simulink model "carBrakeSoln"  (R2015a)
settings: Solver=ode23t  StartTime=0.0  StopTime=50  RelTol=1e-3  AbsTol=1e-3
libraries: nesl_utility x20, fl_lib x18, sdl_lib x11, simulink x1
settings Model: FPTRunName=Active  CovSFcnEnable=off  ExtModeAutoUpdateStatusClock=off  Creator=MathWorks  LastModifiedBy=sseshadr
settings SolverCC: ZcThreshold=0  ZeroCrossAlgorithm=Adaptive
settings DataIOCC: SignalLoggingSaveFormat=ModelDataLogs  SaveOutput=off  SignalLogging=off  DSMLogging=off  SaveTime=off
settings OptimizationCC: ExpressionDepthLimit=2147483647  InitFltsAndDblsToZero=on  BufferReusableBoundary=off
settings DebuggingCC: SaveWithParameterizedLinksMsg=none  UnderspecifiedInitializationDetection=Classic  MergeDetectMultiDrivingBlocksExec=none  SignalResolutionControl=TryResolveAllWithWarning  MultiTaskDSMMsg=warning  MultiTaskCondExecSysMsg=none  SigSpecEnsureSampleTimeMsg=none  FcnCallInpInsideContextMsg=UseLocalSettings  BusObjectLabelMismatch=none  StateNameClashWarn=warning
settings HardwareCC: TargetLongLongMode=on  TargetEndianess=LittleEndian  TargetHWDeviceType=MATLAB Host  ProdEqTarget=off
settings GRTTargetCC: CombineOutputUpdateFcns=off  GRTInterface=on

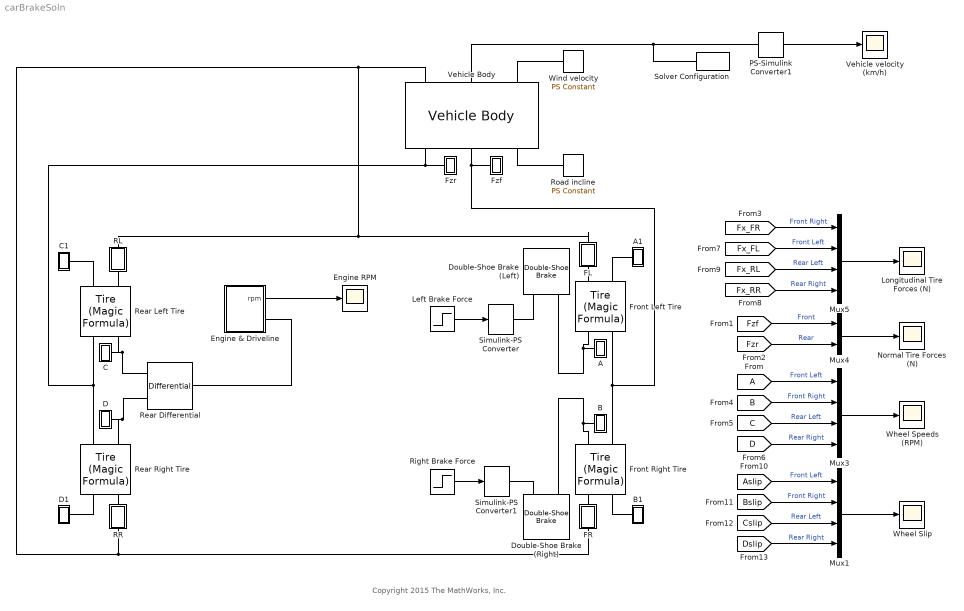
== system carBrakeSoln ==
  note: Copyright 2015 The MathWorks, Inc.
  A : Subsystem
  A1 : Subsystem
  B : Subsystem
  B1 : Subsystem
  C : Subsystem
  C1 : Subsystem
  D : Subsystem
  D1 : Subsystem
  Double-Shoe Brake (Left) : sdl_lib/Brakes & Detents/Rotational/Double-Shoe Brake  r_drum=200 mm  r_act=150 mm  r_pin=125 mm  theta_pin=15 deg  theta_0=5 deg  theta_shoe=120 deg  mu_visc=.01 N*m/(rad/s)  mu=0.3  w_thr=0.01 rad/s
  Double-Shoe Brake (Right) : sdl_lib/Brakes & Detents/Rotational/Double-Shoe Brake  r_drum=200 mm  r_act=150 mm  r_pin=125 mm  theta_pin=15 deg  theta_0=5 deg  theta_shoe=120 deg  mu_visc=.01 N*m/(rad/s)  mu=0.3  w_thr=0.01 rad/s
  Engine RPM : Scope
      settings: TimeRange=30  YMin=600  YMax=1800  SaveName=ScopeData3
  Engine & Driveline : Subsystem
  FL : Subsystem
  FR : Subsystem
  Front Left Tire : sdl_lib/Tires & Vehicles/Tire (Magic Formula)  parameterization=1  F_z1=3000 N  F_x1=3500 N  kappa1=10  B_m=10  C_m=1.9  D_m=1  E_m=0.97  fz0=4e+3 N  p_Cx=1.685  p_Dx=[ 1.21 -0.037 ]  p_Ex=[ 0.344 0.095 -0.02 0 ]  p_Kx=[ 21.51 -0.163 0.245 ]  p_Hx=[ -0.002 0.002 ]  p_Vx=[ 0 0 ]  v_tr_thr=0.1 m/s  r_e=16*2.54/100 m  model_compliance=1  stiffness=200000 N/m  damping=1000 N/(m/s)  model_inertia=1  inertia=4.129 kg*m^2  initial_velocity=0 rpm  model_resistance=1  resistance_model=1  coeff=0.015  p_tire=250e3 Pa  alpha=-0.003  beta=0.97  coeff_a=84e-4  coeff_b=6.2e-4 s/m  coeff_c=1.6e-4 s^2/m^2  v_thr=1e-3 m/s
  Front Right Tire : sdl_lib/Tires & Vehicles/Tire (Magic Formula)  parameterization=1  F_z1=3000 N  F_x1=3500 N  kappa1=10  B_m=10  C_m=1.9  D_m=1  E_m=0.97  fz0=4e+3 N  p_Cx=1.685  p_Dx=[ 1.21 -0.037 ]  p_Ex=[ 0.344 0.095 -0.02 0 ]  p_Kx=[ 21.51 -0.163 0.245 ]  p_Hx=[ -0.002 0.002 ]  p_Vx=[ 0 0 ]  v_tr_thr=0.1 m/s  r_e=16*2.54/100 m  model_compliance=1  stiffness=200000 N/m  damping=1000 N/(m/s)  model_inertia=1  inertia=4.129 kg*m^2  initial_velocity=0 rpm  model_resistance=1  resistance_model=1  coeff=0.015  p_tire=250e3 Pa  alpha=-0.003  beta=0.97  coeff_a=84e-4  coeff_b=6.2e-4 s/m  coeff_c=1.6e-4 s^2/m^2  v_thr=1e-3 m/s
  Fzf : Subsystem
  Fzr : Subsystem
  Left Brake Force : Step  Time=30  After=1000  SampleTime=0
      settings: AttributesFormatString=Brake on @ %<Time> s
  Longitudinal Tire Forces (N) : Scope
      settings: ShowLegends=on  TimeRange=50  YMin=-1500  YMax=3500  SaveName=ScopeData4
  Mux1 : Mux
  Mux3 : Mux
  Mux4 : Mux  Inputs=2
  Mux5 : Mux
  Normal Tire Forces (N) : Scope
      settings: ShowLegends=on  TimeRange=50  YMin=3200  YMax=3900  SaveName=ScopeData2
  PS-Simulink Converter1 : nesl_utility/PS-Simulink Converter  PhysicalDomain=network_engine_domain  SubClassName=ps_output  LeftPortType=input  RightPortType=output  PseudoPeriodic=off  Frequencies=[]  Unit=km/hr  AffineConversion=off
  RL : Subsystem
  RR : Subsystem
  Rear Differential : sdl_lib/Gears/Differential  driveshaft_location=2  cd_ratio=4  friction_model=1  efficiency=[ 0.85 0.92 ]  mu_visc=[ 0 0 ] N*m/(rad/s)  w_thr=[ 0.01 0.01 ] rad/s  temperature_TLU=[ 280 300 320 ] K  efficiency_ss_TLU=[ 0.95 0.9 0.85 ]  efficiency_cd_TLU=[ 0.95 0.9 0.85 ]  thermal_mass=50 J/K  T_init=300 K
  Rear Left Tire : sdl_lib/Tires & Vehicles/Tire (Magic Formula)  parameterization=1  F_z1=3000 N  F_x1=3500 N  kappa1=10  B_m=10  C_m=1.9  D_m=1  E_m=0.97  fz0=4e+3 N  p_Cx=1.685  p_Dx=[ 1.21 -0.037 ]  p_Ex=[ 0.344 0.095 -0.02 0 ]  p_Kx=[ 21.51 -0.163 0.245 ]  p_Hx=[ -0.002 0.002 ]  p_Vx=[ 0 0 ]  v_tr_thr=0.1 m/s  r_e=16*2.54/100 m  model_compliance=1  stiffness=200000 N/m  damping=1000 N/(m/s)  model_inertia=1  inertia=4.129 kg*m^2  initial_velocity=0 rpm  model_resistance=1  resistance_model=1  coeff=0.015  p_tire=250e3 Pa  alpha=-0.003  beta=0.97  coeff_a=84e-4  coeff_b=6.2e-4 s/m  coeff_c=1.6e-4 s^2/m^2  v_thr=1e-3 m/s
  Rear Right Tire : sdl_lib/Tires & Vehicles/Tire (Magic Formula)  parameterization=1  F_z1=3000 N  F_x1=3500 N  kappa1=10  B_m=10  C_m=1.9  D_m=1  E_m=0.97  fz0=4e+3 N  p_Cx=1.685  p_Dx=[ 1.21 -0.037 ]  p_Ex=[ 0.344 0.095 -0.02 0 ]  p_Kx=[ 21.51 -0.163 0.245 ]  p_Hx=[ -0.002 0.002 ]  p_Vx=[ 0 0 ]  v_tr_thr=0.1 m/s  r_e=16*2.54/100 m  model_compliance=1  stiffness=200000 N/m  damping=1000 N/(m/s)  model_inertia=1  inertia=4.129 kg*m^2  initial_velocity=0 rpm  model_resistance=1  resistance_model=1  coeff=0.015  p_tire=250e3 Pa  alpha=-0.003  beta=0.97  coeff_a=84e-4  coeff_b=6.2e-4 s/m  coeff_c=1.6e-4 s^2/m^2  v_thr=1e-3 m/s
  Right Brake Force : Step  Time=30  After=1000  SampleTime=0
      settings: AttributesFormatString=Brake on @ %<Time> s
  Road incline : fl_lib/Physical Signals/Sources/PS Constant  constant=pi*15/180
  Simulink-PS Converter : nesl_utility/Simulink-PS Converter  PhysicalDomain=network_engine_domain  SubClassName=ps_input  LeftPortType=input  RightPortType=output  PseudoPeriodic=off  Frequencies=[]  NoiseDistribution=none  NoiseParameters=[]  Unit=1  AffineConversion=off  InputFiltering=off  SimscapeFilterOrder=1  InputFilterTimeConstant=0.001  UdotUserProvided=1
  Simulink-PS Converter1 : nesl_utility/Simulink-PS Converter  PhysicalDomain=network_engine_domain  SubClassName=ps_input  LeftPortType=input  RightPortType=output  PseudoPeriodic=off  Frequencies=[]  NoiseDistribution=none  NoiseParameters=[]  Unit=1  AffineConversion=off  InputFiltering=off  SimscapeFilterOrder=1  InputFilterTimeConstant=0.001  UdotUserProvided=1
  Solver Configuration : nesl_utility/Solver Configuration  PhysicalDomain=network_engine_domain  SubClassName=solver  LeftPortType=input  RightPortType=generic  Accelerate=off  Tones=[]  Harmonics=[]  SimulateNoise=off  Profile=off  UseLocalSampling=off  EnableSwitchedLinearOptims=on  FrequencyDomain=off  UseCCode=off  RelTol=0.001  AbsTol=1e-06  MinStep=1e-09  ToWorkspace=off  RevertToSquareIcSolve=off  NumHomotopyIterations=100  DoDC=off  ResidualTolerance=1e-9  UseLocalSolver=off  LocalSolverChoice=NE_BACKWARD_EULER_ADVANCER  LocalSolverSampleTime=0.1  DoFixedCost=off  MaxNonlinIter=3  MaxModeIter=2  LinearAlgebra=Sparse  DelaysMemoryBudget=1024  AutomaticFiltering=on  FilteringTimeConstant=0.001
  Vehicle Body : sdl_lib/Tires & Vehicles/Vehicle Body  mass=1500 kg  n_w=2  x_f=1.4 m  x_r=1.6 m  y_c=0.5 m  area=3 m^2  Cd=0.4  v0=0 m/s  g=9.81 m/s^2  rho=1.18 kg/m^3
  Vehicle velocity (km/h) : Scope
      settings: TimeRange=50  YMax=25  SaveName=ScopeData6
  Wheel Slip : Scope
      settings: ShowLegends=on  TimeRange=50  YMin=-0.01  YMax=0.035
  Wheel Speeds (RPM) : Scope
      settings: ShowLegends=on  TimeRange=50  YMin=-20  YMax=140
  Wind velocity : fl_lib/Physical Signals/Sources/PS Constant  constant=0
  wires:
  Engine & Driveline/1(rpm) -> Engine RPM/1
  PS-Simulink Converter1/1 -> Vehicle velocity (km/h)/1
  Left Brake Force/1 -> Simulink-PS Converter/1
  Right Brake Force/1 -> Simulink-PS Converter1/1
  Mux5/1 -> Longitudinal Tire Forces (N)/1
  Mux4/1 -> Normal Tire Forces (N)/1
  Mux3/1 -> Wheel Speeds (RPM)/1
  Mux1/1 -> Wheel Slip/1
  [A] -> Mux3/1  "Front Left"
  [B] -> Mux3/2  "Front Right"
  [C] -> Mux3/3  "Rear Left"
  [D] -> Mux3/4  "Rear Right"
  [Fzf] -> Mux4/1  "Front"
  [Fzr] -> Mux4/2  "Rear"
  [Fx_FR] -> Mux5/1  "Front Right"
  [Fx_FL] -> Mux5/2  "Front Left"
  [Fx_RR] -> Mux5/4  "Rear Right"
  [Fx_RL] -> Mux5/3  "Rear Left"
  [Aslip] -> Mux1/1  "Front Left"
  [Bslip] -> Mux1/2  "Front Right"
  [Cslip] -> Mux1/3  "Rear Left"
  [Dslip] -> Mux1/4  "Rear Right"
  connections:
  Rear Differential/RConn1 -- Rear Left Tire/LConn2 -- C/LConn1
  D/LConn1 -- Rear Right Tire/LConn2 -- Rear Differential/RConn2
  A/LConn1 -- Double-Shoe Brake (Left)/LConn2 -- Front Left Tire/LConn2
  FL/RConn1 -- RL/RConn1 -- RR/RConn1 -- FR/RConn1 -- Vehicle Body/LConn1
  Front Right Tire/LConn1 -- Front Left Tire/LConn1 -- Vehicle Body/RConn2 -- Fzf/LConn1
  Vehicle Body/RConn1 -- Fzr/LConn1 -- Rear Right Tire/LConn1 -- Rear Left Tire/LConn1
  Road incline/RConn1 -- Vehicle Body/RConn3
  Wind velocity/RConn1 -- Vehicle Body/LConn3
  Vehicle Body/LConn2 -- PS-Simulink Converter1/LConn1 -- Solver Configuration/RConn1
  Front Right Tire/RConn2 -- FR/LConn1
  Rear Right Tire/RConn2 -- RR/LConn1
  Front Left Tire/RConn2 -- FL/LConn1
  Rear Left Tire/RConn2 -- RL/LConn1
  Front Left Tire/RConn1 -- A1/LConn1
  Front Right Tire/RConn1 -- B1/LConn1
  Rear Right Tire/RConn1 -- D1/LConn1
  Rear Left Tire/RConn1 -- C1/LConn1
  Double-Shoe Brake (Left)/LConn1 -- Simulink-PS Converter/RConn1
  Double-Shoe Brake (Right)/LConn1 -- Simulink-PS Converter1/RConn1
  Engine & Driveline/RConn1 -- Rear Differential/LConn1
  Front Right Tire/LConn2 -- Double-Shoe Brake (Right)/LConn2 -- B/LConn1

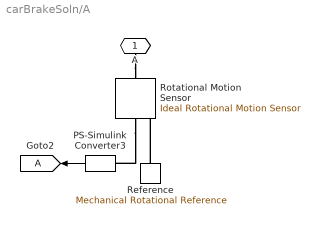
== system carBrakeSoln/A ==
  PS-Simulink Converter3 : nesl_utility/PS-Simulink Converter  PhysicalDomain=network_engine_domain  SubClassName=ps_output  LeftPortType=input  RightPortType=output  PseudoPeriodic=off  Frequencies=[]  Unit=rpm  AffineConversion=off
  Reference : fl_lib/Mechanical/Rotational Elements/Mechanical Rotational Reference
  Rotational Motion Sensor : fl_lib/Mechanical/Mechanical Sensors/Ideal Rotational Motion Sensor  offset=0 rad
  A : PMIOPort  Port=1  Side=Left
  tag scope: A=global
  wires:
  PS-Simulink Converter3/1 -> [A]
  connections:
  Rotational Motion Sensor/RConn2 -- PS-Simulink Converter3/LConn1
  Reference/LConn1 -- Rotational Motion Sensor/RConn1
  A/RConn1 -- Rotational Motion Sensor/LConn1

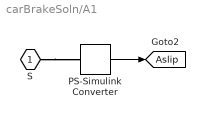
== system carBrakeSoln/A1 ==
  PS-Simulink Converter : nesl_utility/PS-Simulink Converter  PhysicalDomain=network_engine_domain  SubClassName=ps_output  LeftPortType=input  RightPortType=output  PseudoPeriodic=off  Frequencies=[]  Unit=1  AffineConversion=off
  S : PMIOPort  Port=1  Side=Left
  tag scope: Aslip=global
  wires:
  PS-Simulink Converter/1 -> [Aslip]
  connections:
  S/RConn1 -- PS-Simulink Converter/LConn1

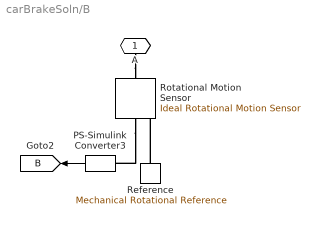
== system carBrakeSoln/B ==
  PS-Simulink Converter3 : nesl_utility/PS-Simulink Converter  PhysicalDomain=network_engine_domain  SubClassName=ps_output  LeftPortType=input  RightPortType=output  PseudoPeriodic=off  Frequencies=[]  Unit=rpm  AffineConversion=off
  Reference : fl_lib/Mechanical/Rotational Elements/Mechanical Rotational Reference
  Rotational Motion Sensor : fl_lib/Mechanical/Mechanical Sensors/Ideal Rotational Motion Sensor  offset=0 rad
  A : PMIOPort  Port=1  Side=Left
  tag scope: B=global
  wires:
  PS-Simulink Converter3/1 -> [B]
  connections:
  A/RConn1 -- Rotational Motion Sensor/LConn1
  Reference/LConn1 -- Rotational Motion Sensor/RConn1
  Rotational Motion Sensor/RConn2 -- PS-Simulink Converter3/LConn1

== system carBrakeSoln/B1 ==
  PS-Simulink Converter : nesl_utility/PS-Simulink Converter  PhysicalDomain=network_engine_domain  SubClassName=ps_output  LeftPortType=input  RightPortType=output  PseudoPeriodic=off  Frequencies=[]  Unit=1  AffineConversion=off
  S : PMIOPort  Port=1  Side=Left
  tag scope: Bslip=global
  wires:
  PS-Simulink Converter/1 -> [Bslip]
  connections:
  S/RConn1 -- PS-Simulink Converter/LConn1

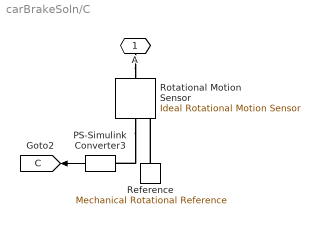
== system carBrakeSoln/C ==
  PS-Simulink Converter3 : nesl_utility/PS-Simulink Converter  PhysicalDomain=network_engine_domain  SubClassName=ps_output  LeftPortType=input  RightPortType=output  PseudoPeriodic=off  Frequencies=[]  Unit=rpm  AffineConversion=off
  Reference : fl_lib/Mechanical/Rotational Elements/Mechanical Rotational Reference
  Rotational Motion Sensor : fl_lib/Mechanical/Mechanical Sensors/Ideal Rotational Motion Sensor  offset=0 rad
  A : PMIOPort  Port=1  Side=Left
  tag scope: C=global
  wires:
  PS-Simulink Converter3/1 -> [C]
  connections:
  Rotational Motion Sensor/RConn2 -- PS-Simulink Converter3/LConn1
  Reference/LConn1 -- Rotational Motion Sensor/RConn1
  A/RConn1 -- Rotational Motion Sensor/LConn1

== system carBrakeSoln/C1 ==
  PS-Simulink Converter : nesl_utility/PS-Simulink Converter  PhysicalDomain=network_engine_domain  SubClassName=ps_output  LeftPortType=input  RightPortType=output  PseudoPeriodic=off  Frequencies=[]  Unit=1  AffineConversion=off
  S : PMIOPort  Port=1  Side=Left
  tag scope: Cslip=global
  wires:
  PS-Simulink Converter/1 -> [Cslip]
  connections:
  S/RConn1 -- PS-Simulink Converter/LConn1

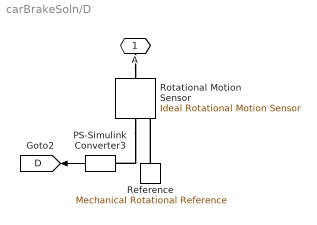
== system carBrakeSoln/D ==
  PS-Simulink Converter3 : nesl_utility/PS-Simulink Converter  PhysicalDomain=network_engine_domain  SubClassName=ps_output  LeftPortType=input  RightPortType=output  PseudoPeriodic=off  Frequencies=[]  Unit=rpm  AffineConversion=off
  Reference : fl_lib/Mechanical/Rotational Elements/Mechanical Rotational Reference
  Rotational Motion Sensor : fl_lib/Mechanical/Mechanical Sensors/Ideal Rotational Motion Sensor  offset=0 rad
  A : PMIOPort  Port=1  Side=Left
  tag scope: D=global
  wires:
  PS-Simulink Converter3/1 -> [D]
  connections:
  A/RConn1 -- Rotational Motion Sensor/LConn1
  Reference/LConn1 -- Rotational Motion Sensor/RConn1
  Rotational Motion Sensor/RConn2 -- PS-Simulink Converter3/LConn1

== system carBrakeSoln/D1 ==
  PS-Simulink Converter : nesl_utility/PS-Simulink Converter  PhysicalDomain=network_engine_domain  SubClassName=ps_output  LeftPortType=input  RightPortType=output  PseudoPeriodic=off  Frequencies=[]  Unit=1  AffineConversion=off
  S : PMIOPort  Port=1  Side=Left
  tag scope: Dslip=global
  wires:
  PS-Simulink Converter/1 -> [Dslip]
  connections:
  S/RConn1 -- PS-Simulink Converter/LConn1

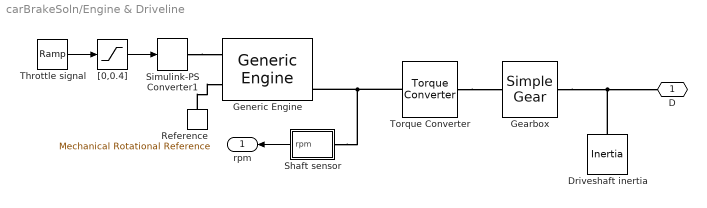
== system carBrakeSoln/Engine & Driveline ==
  Driveshaft inertia : fl_lib/Mechanical/Rotational Elements/Inertia  inertia=12 kg*m^2  w_specify=off  w_priority=High  w=0 rad/s  t_specify=off  t_priority=High  t=0 N*m
  Gearbox : sdl_lib/Gears/Simple Gear  ratio=2  rotation_direction=1  friction_model=1  T_noload=0.1 N*m  T_nom=5 N*m  efficiency_nom=0.8  efficiency=0.8  mu_visc=[ 0 0 ] N*m/(rad/s)  w_thr=0.01 rad/s  temperature_TLU=[ 280 300 320 ] K  load_TLU=[ 1 5 10 ] N*m  efficiency_TLU=[ 0.95 0.9 0.85 ]  efficiency_TLU2=[ 0.85 0.8 0.75; 0.95 0.9 0.85; 0.85 0.8 0.7 ]  thermal_mass=50 J/K  T_init=300 K
  Generic Engine : sdl_lib/Engines/Generic Engine  model_parameterization=1  engine_type=1  P_max=150e3 W  w_P_max=4500 rpm  w_max=6000 rpm  w_min=500 rpm  w_tab=[ 500 1000 2e+3 3e+3 4e+3 5e+3 6e+3 7e+3 ] rpm  trq_tab=[ 380 380 380 380 350 280 200 80 ] N*m  pwr_tab=[ 2e+4 4e+4 7.8e+4 1.2e+5 1.45e+5 1.48e+5 1.25e+5 6e+4 ] W  interp_method=1  model_inertia=1  inertia=0.2 kg*m^2  initial_velocity=800 rpm  model_time_constant=0  time_constant=0.2 s  T0=0  w_thr=100 rpm  idle_speed=0  idle_speed_reference=1000 rpm  tau_controller=1 s  idle_w_thr=1 rpm  fc_model=1  fc_per_rev=25 mg/rev  displaced_volume=400 cm^3  rev_per_cycle=2  fc_w_tab=[ 1000 2e+3 3e+3 4e+3 5e+3 6e+3 ] rpm  fc_trq_tab=[ 0 80 160 200 240 320 360 400 ] N*m  fc_tab=[ 0.5 0.9 1.4 1.6 1.9 2.7 3.4 4.4; 1 1.7 2.7 3.1 3.6 5 6 7.4; 1.4 2.7 4 4.8 5.6 7.5 8.5 10.5; 2 3.6 5.8 6.7 8 10.4 11.7 13.3; 2.5 4.8 7.9 9.4 10.8 14 16.2 18.6; 3.1 6 10.3 11.9 13.8 18.4 22 26.5 ] g/s  bmep_tab=[ 0 250 500 625 750 1000 1.15e+3 1.25e+3 ] kPa  bsfc_tab=[ 410 380 300 280 270 290 320 380; 410 370 290 270 260 270 285 320; 415 380 290 275 265 270 270 300; 420 390 310 290 285 280 280 285; 430 410 340 320 310 300 310 320; 450 430 370 340 330 330 350 380 ] g/hr/kW  fc_interp_method=1
  Reference : fl_lib/Mechanical/Rotational Elements/Mechanical Rotational Reference
  Shaft sensor : Subsystem
  Simulink-PS Converter1 : nesl_utility/Simulink-PS Converter  PhysicalDomain=network_engine_domain  SubClassName=ps_input  LeftPortType=input  RightPortType=output  PseudoPeriodic=off  Frequencies=[]  NoiseDistribution=none  NoiseParameters=[]  Unit=1  AffineConversion=off  InputFiltering=off  SimscapeFilterOrder=1  InputFilterTimeConstant=.001  UdotUserProvided=0
  Throttle signal : simulink/Sources/Ramp  slope=0.9/2  start=0  X0=0.02
  Torque Converter : sdl_lib/Couplings & Drives/Torque Converter  n_vector=[0 0.50 0.60 0.70 0.80 0.87 0.92 0.94 0.96 0.97]  trq_vector=[2.2320 1.5462 1.4058 1.2746 1.1528 1.0732 1.0192 0.9983 0.9983 0.9983]  cf_vector_parameterization=1  cf_vector_reference_speed=1  cf_vector=[12.2938 12.8588 13.1452 13.6285 14.6163 16.2675 19.3503 22.1046 29.9986 50.00] (rad/s)/(N*m)^0.5  cf_vector_sq=1e-3*[ 6.616 6.048 5.787 5.384 4.681 3.779 2.671 2.047 1.111 0.400] N*m/(rad/s)^2  interp_method=1  extrap_method=1  model_lag=0  tau=0.02 s  initial_trq_ratio=0
  "[0,0.4]" : Saturate  UpperLimit=0.4  LowerLimit=0
  D : PMIOPort  Port=1  Side=Right
  rpm : Outport
  wires:
  Shaft sensor/1(rpm) -> rpm/1
  Throttle signal/1 -> "[0,0.4]"/1
  "[0,0.4]"/1 -> Simulink-PS Converter1/1
  connections:
  Torque Converter/LConn1 -- Shaft sensor/LConn1 -- Generic Engine/RConn3
  Reference/LConn1 -- Generic Engine/LConn2
  Simulink-PS Converter1/RConn1 -- Generic Engine/LConn1
  Driveshaft inertia/LConn1 -- D/RConn1 -- Gearbox/RConn1
  Torque Converter/RConn1 -- Gearbox/LConn1

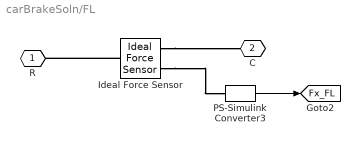
== system carBrakeSoln/FL ==
  Ideal Force Sensor : fl_lib/Mechanical/Mechanical Sensors/Ideal Force Sensor
  PS-Simulink Converter3 : nesl_utility/PS-Simulink Converter  PhysicalDomain=network_engine_domain  SubClassName=ps_output  LeftPortType=input  RightPortType=output  PseudoPeriodic=off  Frequencies=[]  Unit=N  AffineConversion=off
  R : PMIOPort  Port=1  Side=Left
  C : PMIOPort  Port=2  Side=Right
  tag scope: Fx_FL=global
  wires:
  PS-Simulink Converter3/1 -> [Fx_FL]
  connections:
  Ideal Force Sensor/LConn1 -- R/RConn1
  Ideal Force Sensor/RConn1 -- C/RConn1
  Ideal Force Sensor/RConn2 -- PS-Simulink Converter3/LConn1

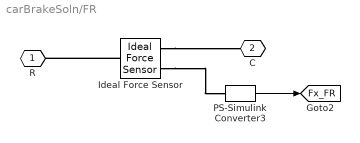
== system carBrakeSoln/FR ==
  Ideal Force Sensor : fl_lib/Mechanical/Mechanical Sensors/Ideal Force Sensor
  PS-Simulink Converter3 : nesl_utility/PS-Simulink Converter  PhysicalDomain=network_engine_domain  SubClassName=ps_output  LeftPortType=input  RightPortType=output  PseudoPeriodic=off  Frequencies=[]  Unit=N  AffineConversion=off
  R : PMIOPort  Port=1  Side=Left
  C : PMIOPort  Port=2  Side=Right
  tag scope: Fx_FR=global
  wires:
  PS-Simulink Converter3/1 -> [Fx_FR]
  connections:
  Ideal Force Sensor/RConn2 -- PS-Simulink Converter3/LConn1
  Ideal Force Sensor/RConn1 -- C/RConn1
  Ideal Force Sensor/LConn1 -- R/RConn1

== system carBrakeSoln/Fzf ==
  PS-Simulink Converter3 : nesl_utility/PS-Simulink Converter  PhysicalDomain=network_engine_domain  SubClassName=ps_output  LeftPortType=input  RightPortType=output  PseudoPeriodic=off  Frequencies=[]  Unit=N  AffineConversion=off
  f : PMIOPort  Port=1  Side=Left
  tag scope: Fzf=global
  wires:
  PS-Simulink Converter3/1 -> [Fzf]
  connections:
  f/RConn1 -- PS-Simulink Converter3/LConn1

== system carBrakeSoln/Fzr ==
  PS-Simulink Converter3 : nesl_utility/PS-Simulink Converter  PhysicalDomain=network_engine_domain  SubClassName=ps_output  LeftPortType=input  RightPortType=output  PseudoPeriodic=off  Frequencies=[]  Unit=N  AffineConversion=off
  f : PMIOPort  Port=1  Side=Left
  tag scope: Fzr=global
  wires:
  PS-Simulink Converter3/1 -> [Fzr]
  connections:
  f/RConn1 -- PS-Simulink Converter3/LConn1

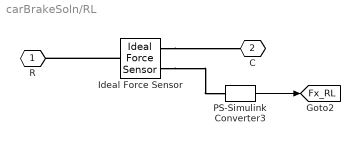
== system carBrakeSoln/RL ==
  Ideal Force Sensor : fl_lib/Mechanical/Mechanical Sensors/Ideal Force Sensor
  PS-Simulink Converter3 : nesl_utility/PS-Simulink Converter  PhysicalDomain=network_engine_domain  SubClassName=ps_output  LeftPortType=input  RightPortType=output  PseudoPeriodic=off  Frequencies=[]  Unit=N  AffineConversion=off
  R : PMIOPort  Port=1  Side=Left
  C : PMIOPort  Port=2  Side=Right
  tag scope: Fx_RL=global
  wires:
  PS-Simulink Converter3/1 -> [Fx_RL]
  connections:
  Ideal Force Sensor/RConn2 -- PS-Simulink Converter3/LConn1
  Ideal Force Sensor/RConn1 -- C/RConn1
  Ideal Force Sensor/LConn1 -- R/RConn1

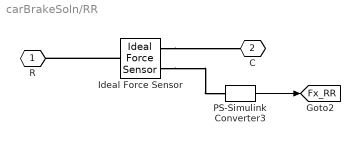
== system carBrakeSoln/RR ==
  Ideal Force Sensor : fl_lib/Mechanical/Mechanical Sensors/Ideal Force Sensor
  PS-Simulink Converter3 : nesl_utility/PS-Simulink Converter  PhysicalDomain=network_engine_domain  SubClassName=ps_output  LeftPortType=input  RightPortType=output  PseudoPeriodic=off  Frequencies=[]  Unit=N  AffineConversion=off
  R : PMIOPort  Port=1  Side=Left
  C : PMIOPort  Port=2  Side=Right
  tag scope: Fx_RR=global
  wires:
  PS-Simulink Converter3/1 -> [Fx_RR]
  connections:
  Ideal Force Sensor/LConn1 -- R/RConn1
  Ideal Force Sensor/RConn1 -- C/RConn1
  Ideal Force Sensor/RConn2 -- PS-Simulink Converter3/LConn1

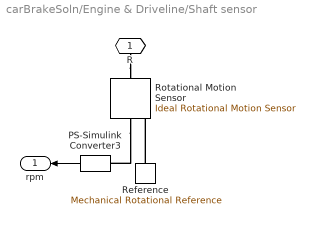
== system carBrakeSoln/Engine & Driveline/Shaft sensor ==
  PS-Simulink Converter3 : nesl_utility/PS-Simulink Converter  PhysicalDomain=network_engine_domain  SubClassName=ps_output  LeftPortType=input  RightPortType=output  PseudoPeriodic=off  Frequencies=[]  Unit=rpm  AffineConversion=off
  Reference : fl_lib/Mechanical/Rotational Elements/Mechanical Rotational Reference
  Rotational Motion Sensor : fl_lib/Mechanical/Mechanical Sensors/Ideal Rotational Motion Sensor  offset=0 rad
  R : PMIOPort  Port=1  Side=Left
  rpm : Outport
  wires:
  PS-Simulink Converter3/1 -> rpm/1
  connections:
  R/RConn1 -- Rotational Motion Sensor/LConn1
  Reference/LConn1 -- Rotational Motion Sensor/RConn1
  Rotational Motion Sensor/RConn2 -- PS-Simulink Converter3/LConn1
